simulink model "second_order"  (R2021a)
settings: Solver=VariableStepAuto  StartTime=0.0  StopTime=1  RelTol=1e-3
libraries: simulink x1
settings Model: Creator=Steven  LastModifiedBy=Steven

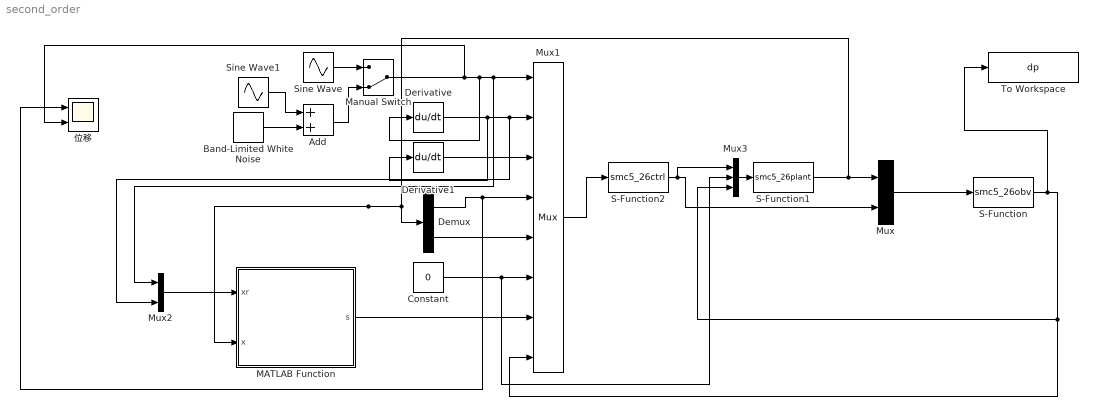
== system second_order ==
  Add : Sum
  Band-Limited White Noise : simulink/Sources/Band-Limited White Noise  Cov=[1e-5*1e-5*0.1]  Ts=0.1  seed=[0]
  Constant : Constant  Value=0
  Demux : Demux  Outputs=2
  Derivative : Derivative
  Derivative1 : Derivative
  MATLAB Function : MATLAB Function  TreatAsAtomicUnit=on
  Manual Switch : ManualSwitch  CurrentSetting=0
  Mux : Mux  Inputs=2
  Mux1 : Mux  Inputs=8
  Mux2 : Mux  Inputs=2
  Mux3 : Mux  Inputs=3
  S-Function : S-Function  FunctionName=smc5_26obv  SFunctionDeploymentMode=off  EnableBusSupport=off
  S-Function1 : S-Function  FunctionName=smc5_26plant  SFunctionDeploymentMode=off  EnableBusSupport=off
  S-Function2 : S-Function  FunctionName=smc5_26ctrl  SFunctionDeploymentMode=off  EnableBusSupport=off
  Sine Wave : Sin  Amplitude=1e-4  Frequency=30*pi  SampleTime=0
  Sine Wave1 : Sin  Amplitude=1e-4  Frequency=30*pi  SampleTime=0
  To Workspace : ToWorkspace  VariableName=dp  SampleTime=-1
      settings: Save2DSignal=2-D array (concatenate along first dimension)
  位移 : Scope  NumInputPorts=2
  wires:
  S-Function1/1 -> Demux/1, MATLAB Function/2(x), Mux/1
  S-Function2/1 -> Mux3/1, Mux/2
  Mux/1 -> S-Function/1
  Mux1/1 -> S-Function2/1
  S-Function/1 -> To Workspace/1, Mux3/3, Mux1/8
  Manual Switch/1 -> 位移/2, Derivative/1, Mux2/1, Mux1/1
  Derivative/1 -> Derivative1/1, Mux2/2, Mux1/2
  Derivative1/1 -> Mux1/3
  Demux/1 -> 位移/1, Mux1/4
  Demux/2 -> Mux1/5
  Constant/1 -> Mux3/2, Mux1/6
  MATLAB Function/1(s) -> Mux1/7
  Mux2/1 -> MATLAB Function/1(xr)
  Mux3/1 -> S-Function1/1
  Sine Wave/1 -> Manual Switch/1
  Add/1 -> Manual Switch/2
  Band-Limited White Noise/1 -> Add/2
  Sine Wave1/1 -> Add/1

== matlab function second_order/MATLAB Function ==
  data: xr input; s output; x input
function s = S(xr,x)
c1 =450;
s = c1*(xr(1)-x(1)) + (xr(2)-x(2));
